simulink model "CBB_ccontrol_pspiceLIN"  (R2021a)
settings: Solver=VariableStepAuto  StartTime=0.0  StopTime=0.2  RelTol=1e-3
undefined symbols (not defined in the file): k, ki, kp, L, R
libraries: pspsim x1, spsSawtoothGeneratorLib x1
settings Model: Creator=Omar_Chavez  LastModifiedBy=omar_

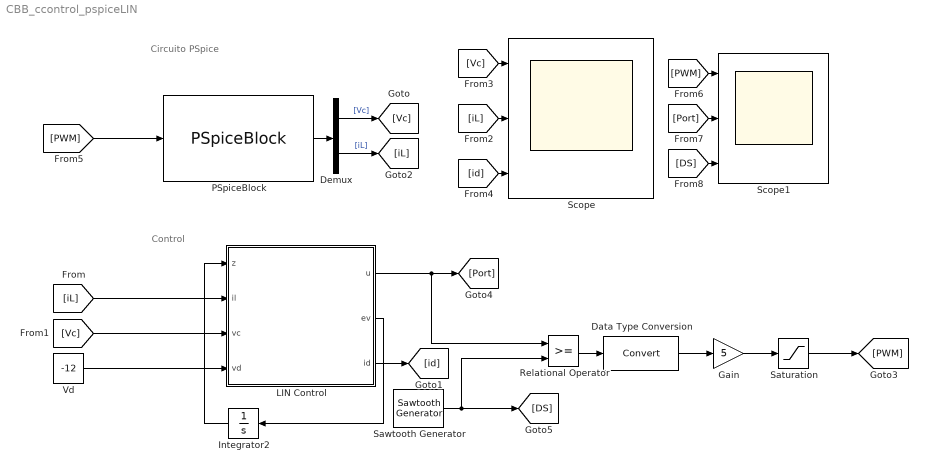
== system CBB_ccontrol_pspiceLIN ==
  note: Control
  note: Circuito PSpice
  Data Type Conversion : DataTypeConversion
  Demux : Demux  Outputs=2
  Gain : Gain  Gain=5
  Integrator2 : Integrator  InitialCondition=0.001
  LIN Control : MATLAB Function  TreatAsAtomicUnit=on
  PSpiceBlock : pspsim/PSpiceBlock  SFunctionModules=''
      settings: SourceProductName=PSpice Block
  Relational Operator : RelationalOperator  OutDataTypeStr=boolean  RndMeth=Simplest
  Saturation : Saturate  UpperLimit=5  LowerLimit=0
  Sawtooth Generator : spsSawtoothGeneratorLib/Sawtooth Generator  Freq=50000  Phase=0  Ts=0
  Scope : Scope  NumInputPorts=3
  Scope1 : Scope  NumInputPorts=3
  Vd : Constant  Value=-12
  wires:
  Sawtooth Generator/1 -> [DS], Relational Operator/2
  Integrator2/1 -> LIN Control/1(z)
  Data Type Conversion/1 -> Gain/1
  Relational Operator/1 -> Data Type Conversion/1
  Gain/1 -> Saturation/1
  LIN Control/2(ev) -> Integrator2/1
  Vd/1 -> LIN Control/4(vd)
  Demux/1 -> [Vc]  "[Vc]"
  Demux/2 -> [iL]  "[iL]"
  LIN Control/3(id) -> [id]
  PSpiceBlock/1 -> Demux/1
  [Vc] -> LIN Control/3(vc)
  [iL] -> LIN Control/2(il)
  [iL] -> Scope/2
  [Vc] -> Scope/1
  [id] -> Scope/3
  Saturation/1 -> [PWM]
  [PWM] -> PSpiceBlock/1
  [PWM] -> Scope1/1
  LIN Control/1(u) -> [Port], Relational Operator/1
  [Port] -> Scope1/2
  [DS] -> Scope1/3

== matlab function CBB_ccontrol_pspiceLIN/LIN Control ==
  data: E parameter; u output; ki parameter; R parameter; kp parameter; k parameter; z input; il input; vc input; L parameter; vd input; ev output; id output
function [u,ev,id] = fcn(E, ki, R, kp, k, z,il,vc,L, vd)

il = double(il); vc = double(vc); 
ev = double(vc -vd);    
id=kp*ev+ki*z;
u=(-vc-k*L*(il-id))/(E-vc);
